simulink model "Amplifi"  (R2024b)
settings: Solver=VariableStepAuto  StartTime=0.0  StopTime=0.003  RelTol=1e-3
values from neighbouring files (symbols this model uses):
  b = (R3+R4)/R3    (= 2.5)    [Amplificadores.m]
  C1 = 1e-7    (= 1e-07)    [Amp.m]    (also in Amplificadores.m)
  C2 = 1e-7    (= 1e-07)    [Amp.m]    (also in Amplificadores.m)
  R1 = 1000    [Amp.m]    (also in Amplificadores.m)
  R2 = 1000    [Amp.m]    (also in Amplificadores.m)
  R3 = 10000    [Amp.m]    (also in Amplificadores.m)
  R4 = 15000    [Amp.m]    (also in Amplificadores.m)
libraries: fl_lib x12, nesl_utility x3
settings Model: Creator=PC  LastModifiedBy=Carlos Iñiguez
settings OptimizationCC: ReuseModelBlockBuffer=off
settings RTWCC: GPUComputeCapability=3.5

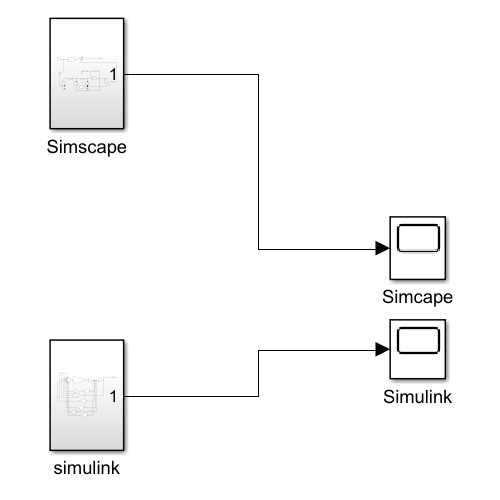
[thumbnail: Simulink's stored preview of the top-level diagram]
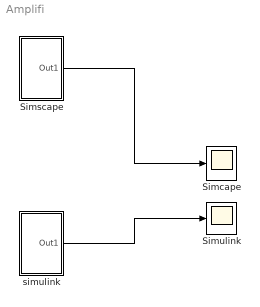
== system Amplifi ==
  Simcape : Scope
  Simscape : Subsystem
  Simulink : Scope
  simulink : Subsystem
  wires:
  Simscape/1(Out1) -> Simcape/1
  simulink/1(Out1) -> Simulink/1

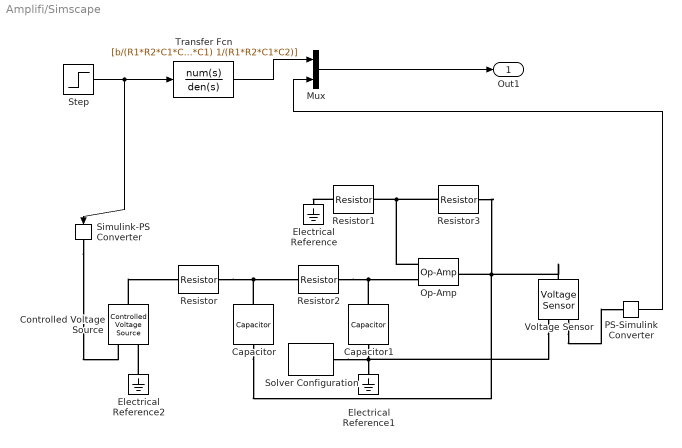
== system Amplifi/Simscape ==
  Capacitor : fl_lib/Electrical/Electrical Elements/Capacitor  c=0.1 uF  r=1e-6 Ohm  g=0 1/Ohm  i_specify=off  i_priority=None  i=0 A  i_nominal_specify=off  i_nominal_value=1  i_nominal_unit=A  v_specify=off  v_priority=None  v=0 V  v_nominal_specify=off  v_nominal_value=1  v_nominal_unit=V  vc_specify=off  vc_priority=High  vc=0 V  vc_nominal_specify=off  vc_nominal_value=1  vc_nominal_unit=V
  Capacitor1 : fl_lib/Electrical/Electrical Elements/Capacitor  c=0.1 uF  r=1e-6 Ohm  g=0 1/Ohm  i_specify=off  i_priority=None  i=0 A  i_nominal_specify=off  i_nominal_value=1  i_nominal_unit=A  v_specify=off  v_priority=None  v=0 V  v_nominal_specify=off  v_nominal_value=1  v_nominal_unit=V  vc_specify=off  vc_priority=High  vc=0 V  vc_nominal_specify=off  vc_nominal_value=1  vc_nominal_unit=V
  Controlled Voltage Source : fl_lib/Electrical/Electrical Sources/Controlled Voltage Source
  Electrical Reference : fl_lib/Electrical/Electrical Elements/Electrical Reference
  Electrical Reference1 : fl_lib/Electrical/Electrical Elements/Electrical Reference
  Electrical Reference2 : fl_lib/Electrical/Electrical Elements/Electrical Reference
  Mux : Mux  Inputs=2
  Op-Amp : fl_lib/Electrical/Electrical Elements/Op-Amp  outI_specify=off  outI_priority=None  outI=0 A  outI_nominal_specify=off  outI_nominal_value=1  outI_nominal_unit=A
  PS-Simulink Converter : nesl_utility/PS-Simulink Converter  PhysicalDomain=network_engine_domain  SubClassName=ps_output  LeftPortType=input  RightPortType=output  PseudoPeriodic=off  Frequencies=[]  VectorFormat=inherit  Unit=inherit  AffineConversion=off
  Resistor : fl_lib/Electrical/Electrical Elements/Resistor  R=1 kOhm  i_specify=off  i_priority=None  i=0 A  i_nominal_specify=off  i_nominal_value=1  i_nominal_unit=A  v_specify=off  v_priority=None  v=0 V  v_nominal_specify=off  v_nominal_value=1  v_nominal_unit=V
  Resistor1 : fl_lib/Electrical/Electrical Elements/Resistor  R=10 kOhm  i_specify=off  i_priority=None  i=0 A  i_nominal_specify=off  i_nominal_value=1  i_nominal_unit=A  v_specify=off  v_priority=None  v=0 V  v_nominal_specify=off  v_nominal_value=1  v_nominal_unit=V
  Resistor2 : fl_lib/Electrical/Electrical Elements/Resistor  R=1 kOhm  i_specify=off  i_priority=None  i=0 A  i_nominal_specify=off  i_nominal_value=1  i_nominal_unit=A  v_specify=off  v_priority=None  v=0 V  v_nominal_specify=off  v_nominal_value=1  v_nominal_unit=V
  Resistor3 : fl_lib/Electrical/Electrical Elements/Resistor  R=15 kOhm  i_specify=off  i_priority=None  i=0 A  i_nominal_specify=off  i_nominal_value=1  i_nominal_unit=A  v_specify=off  v_priority=None  v=0 V  v_nominal_specify=off  v_nominal_value=1  v_nominal_unit=V
  Simulink-PS Converter : nesl_utility/Simulink-PS Converter  PhysicalDomain=network_engine_domain  SubClassName=ps_input  LeftPortType=input  RightPortType=output  PseudoPeriodic=off  Frequencies=[]  NoiseDistribution=none  NoiseParameters=[]  Unit=1  AffineConversion=off  FilteringAndDerivatives=provide  SimscapeFilterOrder=1  InputFilterTimeConstant=0.001  UdotUserProvided=0
  Solver Configuration : nesl_utility/Solver Configuration  PhysicalDomain=network_engine_domain  SubClassName=solver  LeftPortType=input  RightPortType=generic  Tones=[]  Harmonics=[]  SimulateNoise=off  Profile=off  UseLocalSampling=off  EnableSwitchedLinearOptims=on  FrequencyDomain=off  UseCCode=off  RelTol=0.001  AbsTol=0.001  MinStep=1e-09  ToWorkspace=off  RevertToSquareIcSolve=off  NumHomotopyIterations=100  PhasorMode=off  PhasorModeNumHarmonics=1  ConsistencySolver=NEWTON_XTOL_AFTER_FTOL  IndexReductionMethod=DerivativeReplacement  DoDC=off  ResidualTolerance=1e-09  ConsistencyTolSource=GLOBAL  ConsistencyAbsTol=0.001  ConsistencyRelTol=0.001  ConsistencyTolFactor=0.001  UseLocalSolver=off  LocalSolverChoice=NE_BACKWARD_EULER_ADVANCER  ResolveIndetEquations=on  FunctionEvalNumThread=1  LocalSolverSampleTime=0.001  DoFixedCost=off  MaxNonlinIter=3  MaxModeIter=2  ComputeImpulses=off  ImpulseIterations=2  LinearAlgebra=auto  LinearAlgebraNumThread=0  EquationFormulation=NE_TIME_EF  DelaysMemoryBudget=1024  AutomaticFiltering=on  FilteringTimeConstant=0.001  PartitionStorageMethod=AS_NEEDED  PartitionMemoryBudget=1024  PartitionMethod=ROBUST  MultibodyUseLocalSolver=off  MultibodyLocalSolverChoice=ODE1  MultibodyLocalSolverSampleTime=0.001
  Step : Step  Time=0  Before=1  SampleTime=0
  Transfer Fcn : TransferFcn  Numerator=[b/(R1*R2*C1*C2)]  Denominator=[1 1/(R1*C1)+(1-b)/(R2*C2)+1/(R2*C1) 1/(R1*R2*C1*C2)]
  Voltage Sensor : fl_lib/Electrical/Electrical Sensors/Voltage Sensor
  Out1 : Outport
  wires:
  Mux/1 -> Out1/1
  Transfer Fcn/1 -> Mux/1
  Step/1 -> Simulink-PS Converter/1, Transfer Fcn/1
  PS-Simulink Converter/1 -> Mux/2
  connections:
  Capacitor1/LConn1 -- Op-Amp/LConn1 -- Resistor2/RConn1
  Controlled Voltage Source/LConn1 -- Resistor/LConn1
  Resistor1/LConn1 -- Electrical Reference/LConn1
  Capacitor1/RConn1 -- Solver Configuration/RConn1 -- Voltage Sensor/RConn2 -- Electrical Reference1/LConn1
  Simulink-PS Converter/RConn1 -- Controlled Voltage Source/RConn1
  Op-Amp/LConn2 -- Resistor3/LConn1 -- Resistor1/RConn1
  Resistor3/RConn1 -- Voltage Sensor/LConn1 -- Op-Amp/RConn1 -- Capacitor/LConn1
  Capacitor/RConn1 -- Resistor2/LConn1 -- Resistor/RConn1
  Electrical Reference2/LConn1 -- Controlled Voltage Source/RConn2
  Voltage Sensor/RConn1 -- PS-Simulink Converter/LConn1

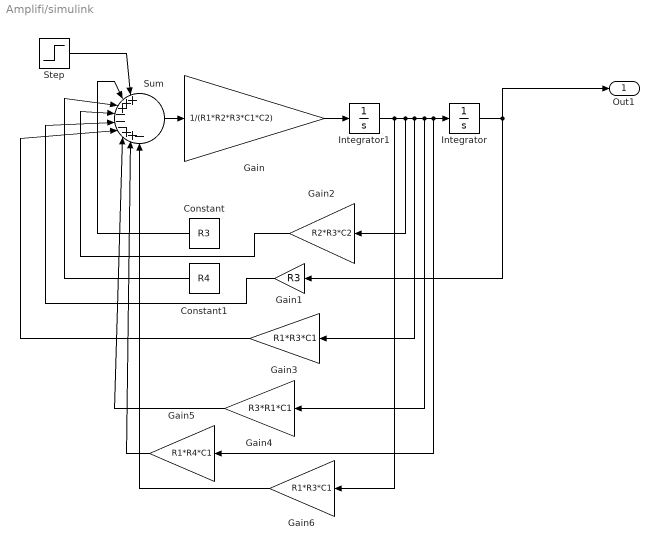
== system Amplifi/simulink ==
  Constant : Constant  Value=R3
  Constant1 : Constant  Value=R4
  Gain : Gain  Gain=1/(R1*R2*R3*C1*C2)
  Gain1 : Gain  Gain=R3
  Gain2 : Gain  Gain=R2*R3*C2
  Gain3 : Gain  Gain=R1*R3*C1
  Gain4 : Gain  Gain=R3*R1*C1
  Gain5 : Gain  Gain=R1*R4*C1
  Gain6 : Gain  Gain=R1*R3*C1
  Integrator : Integrator
  Integrator1 : Integrator
  Step : Step  Time=0  Before=1  SampleTime=0
  Sum : Sum  Inputs=|+++---++-
  Out1 : Outport
  wires:
  Gain1/1 -> Sum/5
  Constant1/1 -> Sum/3
  Integrator1/1 -> Gain6/1, Gain2/1, Gain3/1, Gain4/1, Gain5/1, Integrator/1
  Integrator/1 -> Gain1/1, Out1/1
  Constant/1 -> Sum/2
  Step/1 -> Sum/1
  Gain/1 -> Integrator1/1
  Gain3/1 -> Sum/6
  Sum/1 -> Gain/1
  Gain6/1 -> Sum/9
  Gain4/1 -> Sum/7
  Gain2/1 -> Sum/4
  Gain5/1 -> Sum/8
